simulink model "VisionModel_debugging"  (Simulink 7.6)
settings: Solver=FixedStepDiscrete  StartTime=0.0  StopTime=0  RelTol=1e-3
settings Model: Creator=Administrator  LastModifiedBy=auvt
settings OptimizationCC: OptimizeModelRefInitCode=on
settings RTWCC: SystemTargetFile=ert.tlc  GenCodeOnly=on  TemplateMakefile=ert_default_tmf  PostCodeGenCommand=packNGo(buildInfo, {'packType' 'flat'})  Description=Real-Time Workshop Embedded Coder  GenerateReport=on  ProcessScript=ert_make_rtw_hook  IncludeHyperlinkInReport=on  LaunchReport=on  TargetLang=C++
settings CodeAppCC: IgnoreCustomStorageClasses=off
settings ERTTargetCC: MultiwordLength=2048  GenerateSampleERTMain=on  IncludeMdlTerminateFcn=off  ERTCustomFileTemplate=example_file_process.tlc  ConvertIfToSwitch=off

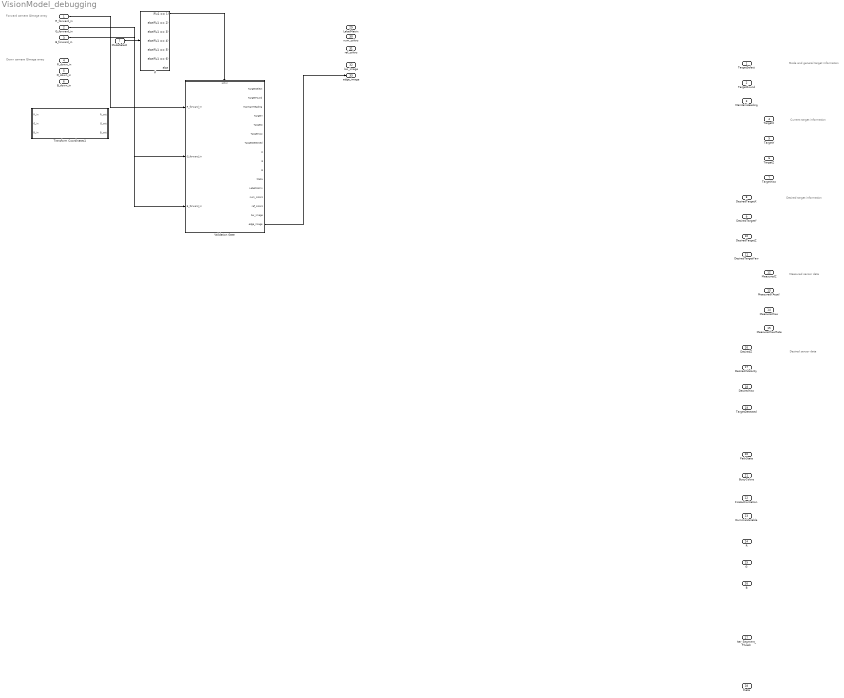
== system VisionModel_debugging ==
  note: Current target information
  note: Desired target information
  note: Measured sensor data
  note: Mode and general target information
  note: Desired sensor data
  note: Forward camera QImage array
  note: Down camera QImage array
  R_forward_in : Inport  PortDimensions=Forward_Camera_Dimensions
  G_forward_in : Inport  Port=2  PortDimensions=Forward_Camera_Dimensions
  B_forward_in : Inport  Port=3  PortDimensions=Forward_Camera_Dimensions
  R_down_in : Inport  Port=4  PortDimensions=Down_Camera_Dimensions
  G_down_in : Inport  Port=5  PortDimensions=Down_Camera_Dimensions
  B_down_in : Inport  Port=6  PortDimensions=Down_Camera_Dimensions
  ModeSelect : Inport  Port=7
  If : If  IfExpression=u1 == 1  ElseIfExpressions=u1 == 2, u1 == 3, u1 == 4, u1 == 5, u1 == 6
  Transform Coordinates1 : Stateflow chart  TreatAsAtomicUnit=on  SystemSampleTime=[1/30 0]
  Validation Gate : Subsystem  TreatAsAtomicUnit=on
  TargetSelect : Outport  OutDataTypeStr=double
  TargetFound : Outport  Port=2  OutDataTypeStr=double
  MaintainHeading : Outport  Port=3  OutDataTypeStr=double
  TargetX : Outport  Port=4  OutDataTypeStr=double
  TargetY : Outport  Port=5  OutDataTypeStr=double
  TargetZ : Outport  Port=6  OutDataTypeStr=double
  TargetYaw : Outport  Port=7  OutDataTypeStr=double
  DesiredTargetX : Outport  Port=8  OutDataTypeStr=double
  DesiredTargetY : Outport  Port=9  OutDataTypeStr=double
  DesiredTargetZ : Outport  Port=10  OutDataTypeStr=double
  DesiredTargetYaw : Outport  Port=11  OutDataTypeStr=double
  MeasuredZ : Outport  Port=12  OutDataTypeStr=double
  MeasuredYAccel : Outport  Port=13  OutDataTypeStr=double
  MeasuredYaw : Outport  Port=14  OutDataTypeStr=double
  MeasuredYawRate : Outport  Port=15  OutDataTypeStr=double
  DesiredZ : Outport  Port=16  OutDataTypeStr=double
  DesiredXVelocity : Outport  Port=17  OutDataTypeStr=double
  DesiredYaw : Outport  Port=18  OutDataTypeStr=double
  TargetDetected : Outport  Port=19  OutDataTypeStr=double
  PathState : Outport  Port=20  OutDataTypeStr=double
  BuoyColors : Outport  Port=21  OutDataTypeStr=double
  FireAuthorization : Outport  Port=22  OutDataTypeStr=double
  DummieVariable : Outport  Port=23  OutDataTypeStr=double
  R : Outport  Port=24  OutDataTypeStr=double
  G : Outport  Port=25  OutDataTypeStr=double
  B : Outport  Port=26  OutDataTypeStr=double
  Iter_Segment_Thresh : Outport  Port=27  OutDataTypeStr=double
  theta : Outport  Port=28  OutDataTypeStr=double
  LabelMatrix : Outport  Port=29
  num_colors : Outport  Port=30
  ref_colors : Outport  Port=31
  bw_image : Outport  Port=32
  edge_image : Outport  Port=33
  wires:
  ModeSelect/1 -> If/1
  If/1 -> Validation Gate/Action
  Validation Gate/16(edge_image) -> edge_image/1
  R_forward_in/1 -> Validation Gate/1(R_forward_in)
  G_forward_in/1 -> Validation Gate/2(G_forward_in)
  B_forward_in/1 -> Validation Gate/3(B_forward_in)

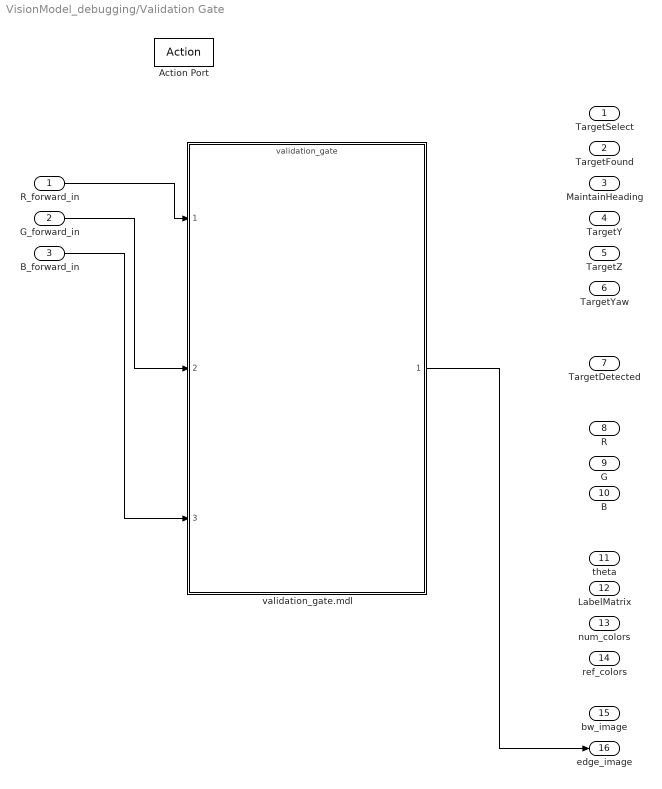
== system VisionModel_debugging/Validation Gate ==
  R_forward_in : Inport
  G_forward_in : Inport  Port=2
  B_forward_in : Inport  Port=3
  Action Port : ActionPort  ActionType=then
  validation_gate.mdl : ModelReference  ModelNameDialog=validation_gate  SimulationMode=Accelerator  ModelReferenceVersion=1.1219  CopyOfModelName=validation_gate
  TargetSelect : Outport  OutDataTypeStr=double
  TargetFound : Outport  Port=2  OutDataTypeStr=double
  MaintainHeading : Outport  Port=3  OutDataTypeStr=double
  TargetY : Outport  Port=4  OutDataTypeStr=double
  TargetZ : Outport  Port=5  OutDataTypeStr=double
  TargetYaw : Outport  Port=6  OutDataTypeStr=double
  TargetDetected : Outport  Port=7  OutDataTypeStr=double
  R : Outport  Port=8  OutDataTypeStr=double
  G : Outport  Port=9  OutDataTypeStr=double
  B : Outport  Port=10  OutDataTypeStr=double
  theta : Outport  Port=11  OutDataTypeStr=double
  LabelMatrix : Outport  Port=12
  num_colors : Outport  Port=13
  ref_colors : Outport  Port=14
  bw_image : Outport  Port=15
  edge_image : Outport  Port=16
  wires:
  R_forward_in/1 -> validation_gate.mdl/1
  G_forward_in/1 -> validation_gate.mdl/2
  B_forward_in/1 -> validation_gate.mdl/3
  validation_gate.mdl/1 -> edge_image/1

== matlab function Transform Coordinates1 ==
  data: R_in input double; G_in input double; R_out output double; G_out output double; B_in input double; B_out output double
function [R_out, G_out, B_out] = rangeImage(R_in, G_in, B_in)
% Ensure the image components are between 0 and newMax

newMax = 1;

R_out = R_in;
G_out = G_in;
B_out = B_in;

normalizeValue = max(max(R_in));
if( normalizeValue <= 1 )
    normalizeValue = 1;
else
    normalizeValue = 255;
end

[rows, cols] = size(R_in);


for r = 1:rows
    for c = 1:cols
        
        if( R_in(r,c) == 0 )
            R_out(r,c) = 0;
        else
            R_out(r,c) = newMax*R_in(r,c)/normalizeValue;
        end
        if( G_in(r,c) == 0 )
            G_out(r,c) = 0;
        else
            G_out(r,c) = newMax*G_in(r,c)/normalizeValue;
        end
        if( B_in(r,c) == 0 )
            B_out(r,c) = 0;
        else
            B_out(r,c) = newMax*B_in(r,c)/normalizeValue;
        end
        
    end
end


return
